simulink model "Ters_Sarkac"  (R2022a)
settings: Solver=ode4  StartTime=0.0  StopTime=10.0  FixedStep=1/1000  RelTol=1e-3
InitFcn:
  | Sarkac_Parametrelerini_Yukle
values from neighbouring files (symbols this model uses):
  b = 0.1    [Sarkac_Parametrelerini_Yukle.m]
  g = 9.8    [Sarkac_Parametrelerini_Yukle.m]
  I = 0.006    [Sarkac_Parametrelerini_Yukle.m]
  l = 0.3    [Sarkac_Parametrelerini_Yukle.m]
  M = 0.5    [Sarkac_Parametrelerini_Yukle.m]
  m = 0.2    [Sarkac_Parametrelerini_Yukle.m]
undefined symbols (not defined in the file or in its folder): sigbuilder_block
libraries: vrlib x1
settings Model: Creator=Fatabi  LastModifiedBy=Fatabi
settings SolverCC: AlgebraicLoopSolver=TrustRegion
settings DebuggingCC: UnconnectedInputMsg=warning  UnconnectedOutputMsg=warning  UnconnectedLineMsg=warning  SFMachineParentedDataDiag=warning

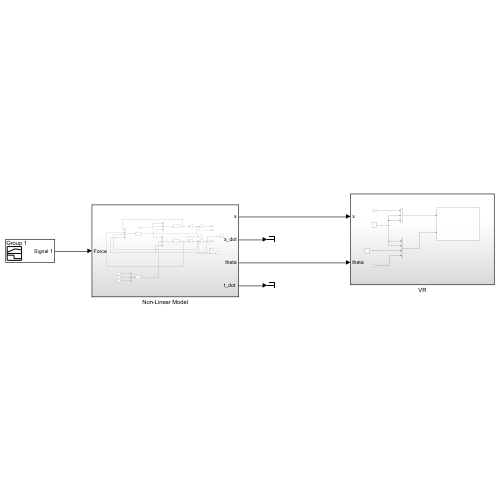
[thumbnail: Simulink's stored preview of the top-level diagram]
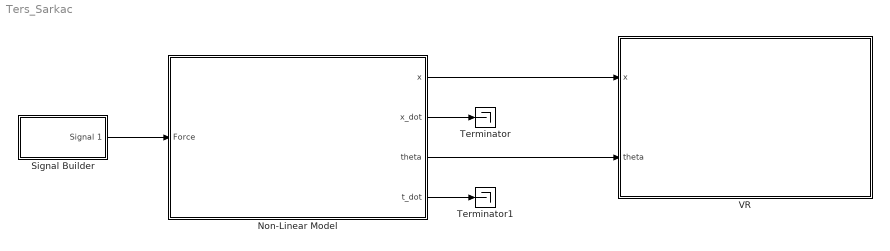
== system Ters_Sarkac ==
  Non-Linear Model : Subsystem
  Signal Builder : Subsystem  Tag=STV Subsys  LoadFcn=sigbuilder_block('load');  StartFcn=sigbuilder_block('start');  StopFcn=sigbuilder_block('stop');  ClipboardFcn=sigbuilder_block('clipboard');  mask(Sigbuilder block){tuvar=[0:10]}
      mask help: Simulink:masks:SigbuilderBlock_MD
      mask init:
      | if ~strcmp(get_param(bdroot(gcbh),'SimulationStatus'),'stopped') tuvar = sigbuilder_block('maskInit'); end
      settings: CopyFcn=sigbuilder_block('copy');  DeleteFcn=sigbuilder_block('delete');  ModelCloseFcn=sigbuilder_block('modelClose');  PreSaveFcn=sigbuilder_block('preSave');  PauseFcn=sigbuilder_block('pause');  ContinueFcn=sigbuilder_block('continue');  NameChangeFcn=sigbuilder_block('namechange');  OpenFcn=sigbuilder_block('open',[338.25 225.75 550.5 399.75 ]);  CloseFcn=sigbuilder_block('close');
      mask Display: plot(0, 0, 100, 100,[2, 2, 32, 32, 2], [68, 8, 8, 68, 68],[32, 2], [38, 38], [32, 19, 2],[53, 60, 44], [32, 17, 17, 2],[16, 16, 31, 31]);txt = getActiveGroup(gcbh);text(2, 100, txt,'verticalAlignment', 'top');
  Terminator : Terminator
  Terminator1 : Terminator
  "VR " : Subsystem
  wires:
  Non-Linear Model/1(x) -> "VR "/1(x)
  Non-Linear Model/3(theta) -> "VR "/2("theta ")
  Non-Linear Model/2(x_dot) -> Terminator/1
  Non-Linear Model/4("t_dot ") -> Terminator1/1
  Signal Builder/1(Signal 1) -> Non-Linear Model/1(Force)

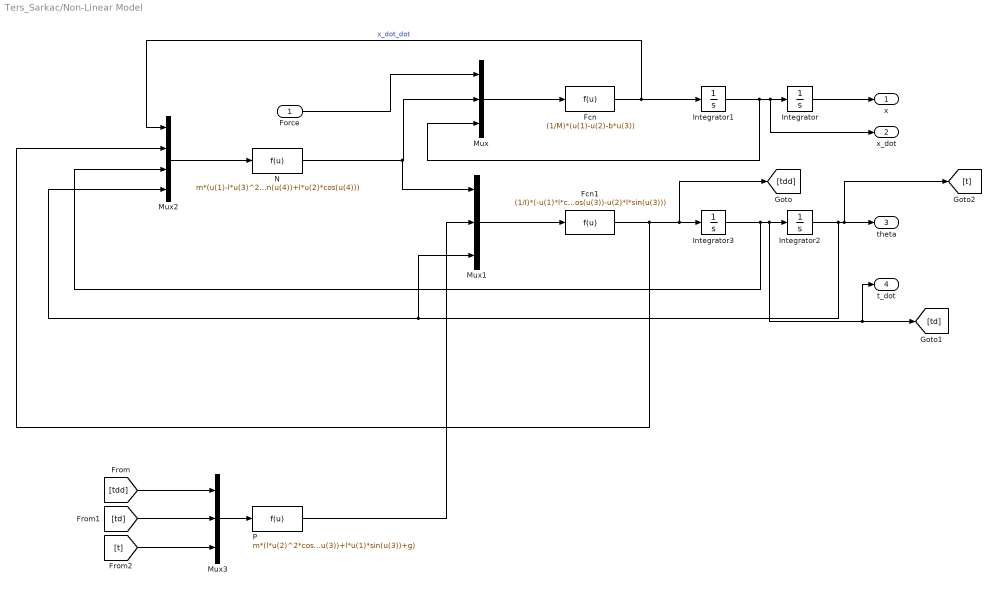
== system Ters_Sarkac/Non-Linear Model ==
  Force : Inport
  Fcn : Fcn  Expr=(1/M)*(u(1)-u(2)-b*u(3))
  Fcn1 : Fcn  Expr=(1/I)*(-u(1)*l*cos(u(3))-u(2)*l*sin(u(3)))
  Integrator : Integrator
  Integrator1 : Integrator
  Integrator2 : Integrator  InitialCondition=pi-0.1
  Integrator3 : Integrator
  Mux : Mux  Inputs=3
  Mux1 : Mux  Inputs=3
  Mux2 : Mux
  Mux3 : Mux  Inputs=3
  N : Fcn  Expr=m*(u(1)-l*u(3)^2*sin(u(4))+l*u(2)*cos(u(4)))
  P : Fcn  Expr=m*(l*u(2)^2*cos(u(3))+l*u(1)*sin(u(3))+g)
  x : Outport
  x_dot : Outport  Port=2
  theta : Outport  Port=3
  "t_dot " : Outport  Port=4
  wires:
  Integrator/1 -> x/1
  Integrator1/1 -> x_dot/1, Integrator/1, Mux/3
  Fcn/1 -> Mux2/1, Integrator1/1  "x_dot_dot"
  Integrator3/1 -> Mux2/3, "t_dot "/1, [td], Integrator2/1
  Integrator2/1 -> Mux2/4, Mux1/3, [t], theta/1
  Force/1 -> Mux/1
  N/1 -> Mux1/1, Mux/2
  Mux/1 -> Fcn/1
  Fcn1/1 -> Mux2/2, [tdd], Integrator3/1
  Mux1/1 -> Fcn1/1
  P/1 -> Mux1/2
  Mux2/1 -> N/1
  [tdd] -> Mux3/1
  [td] -> Mux3/2
  [t] -> Mux3/3
  Mux3/1 -> P/1

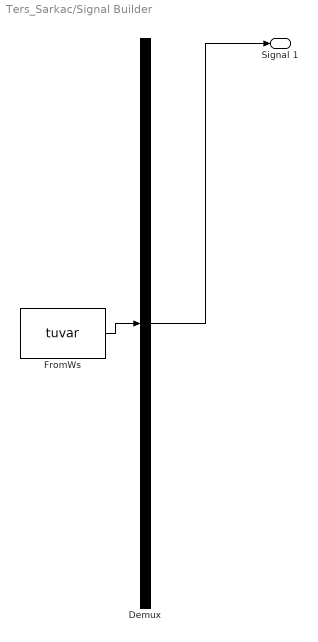
== system Ters_Sarkac/Signal Builder ==
  Demux : Demux  Tag=STV Demux  Outputs=1
      settings: DisplayOption=none
  FromWs : FromWorkspace  Tag=STV FromWs  VariableName=tuvar
      SigBuilderData=|
      | common.afterFinalStr = 'Extrapolate'
      | common.sampleTime = 0
      | dataSet.timeRange = [0 10]
      | dataSet.name = 'Group 1'
      | sbobj.Groups.Name = 'Group 1'
      | sbobj.Groups.Signals.Name = 'Signal 1'
      | sbobj.Groups.Signals.XData = [0 1.04 1.04 1.82 1.82 10]
      | sbobj.Groups.Signals.YData = [0 0 1 1 0 0]
  Signal 1 : Outport  Tag=STV Outport
  wires:
  Demux/1 -> Signal 1/1
  FromWs/1 -> Demux/1

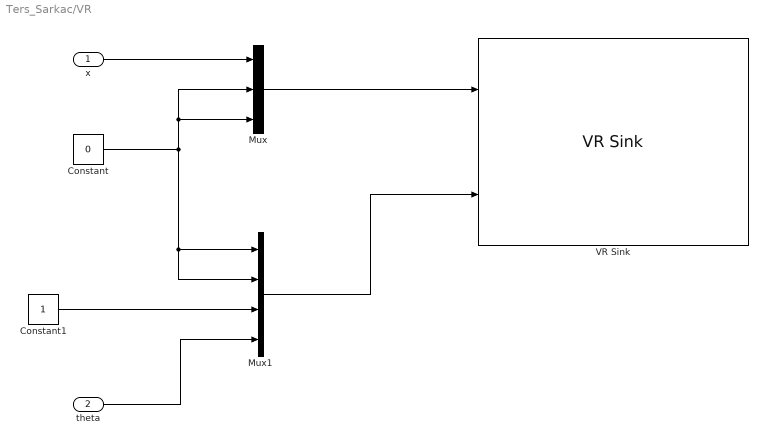
== system Ters_Sarkac/VR  ==
  x : Inport
  "theta " : Inport  Port=2
  Constant : Constant  Value=0
  Constant1 : Constant
  Mux : Mux  Inputs=3
  Mux1 : Mux
  VR Sink : vrlib/VR Sink  InstantiateOnLoad=on  SampleTime=0.02  ViewEnable=on  RemoteChange=off  RemoteView=off  FieldsWritten=Kutu.translation.3.1.1.double#Mentese1.rotation.4.1.1.double  WorldFileName=sarkac.wrl  AutoView=off  VideoDimensions=[]  AllowVariableSize=off
  wires:
  x/1 -> Mux/1
  Constant/1 -> Mux/3, Mux/2, Mux1/2, Mux1/1
  "theta "/1 -> Mux1/4
  Constant1/1 -> Mux1/3
  Mux/1 -> VR Sink/1
  Mux1/1 -> VR Sink/2
